simulink model "AerialManipulatorSystem"  (R2023b)
settings: Solver=FixedStepDiscrete  StartTime=0  StopTime=10  FixedStep=0.01  RelTol=1e-3
settings Model: Creator=Chen Fan  LastModifiedBy=Chen Fan
settings DataIOCC: ReturnWorkspaceOutputs=off

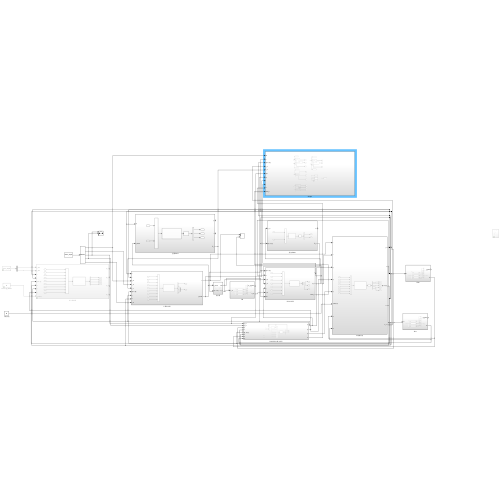
[thumbnail: Simulink's stored preview of the top-level diagram]
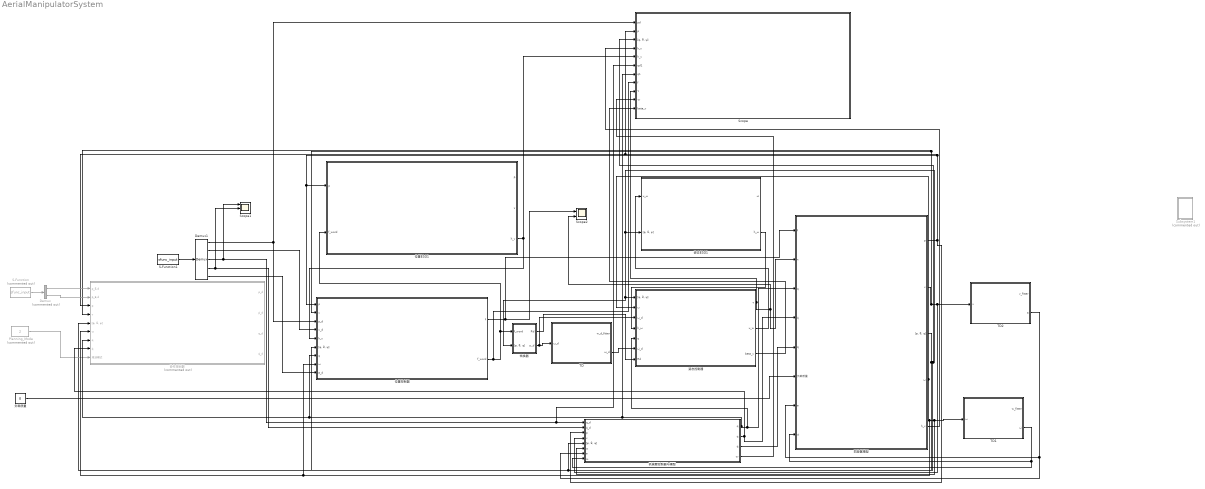
== system AerialManipulatorSystem ==
  Demux : Demux  Commented=on  Outputs=2
  Demux1 : Demux  Outputs=5
      settings: DisplayOption=none
  Planning_Mode : Constant  Commented=on  Value=2
  S-Function : S-Function  Commented=on  FunctionName=sfunc_input  SFunctionDeploymentMode=off  EnableBusSupport=off
  S-Function1 : S-Function  FunctionName=sfunc_input  SFunctionDeploymentMode=off  EnableBusSupport=off
  Scope : Subsystem
  Scope1 : Scope  NumInputPorts=3
  Scope2 : Scope  NumInputPorts=2
  Subsystem1 : Subsystem  Commented=on
  TD : Subsystem
  TD1 : Subsystem
  TD2 : Subsystem
  位置ESO1 : Subsystem
  位置控制器 : Subsystem
  协作规划器 : Subsystem  Commented=on
  四旋翼模型 : Subsystem
  姿态ESO1 : Subsystem
  姿态控制器 : Subsystem
  机械臂控制器与模型 : Subsystem
  负载质量 : Constant  Value=0
  转换器 : Subsystem
  wires:
  姿态控制器/1(τ) -> 四旋翼模型/2(τ), Scope2/2, Scope/9(τ)
  位置控制器/1(f) -> Scope2/1, 四旋翼模型/1(f)
  四旋翼模型/3("[φ, θ, ψ]") -> 位置控制器/6("[φ, θ, ψ]"), 机械臂控制器与模型/5("[φ, θ, ψ]"), 姿态ESO1/2("[φ, θ, ψ]"), 转换器/2("[φ, θ, ψ]"), 姿态控制器/1("[φ, θ, ψ]"), Scope/3("[φ, θ, ψ]"), 协作规划器/5("[φ, θ, ψ]")
  负载质量/1 -> 四旋翼模型/6(负载质量)
  四旋翼模型/1(p) -> 机械臂控制器与模型/3(p), 位置ESO1/1(p), 位置控制器/1(p), 协作规划器/3(p), Scope/2(p)
  Planning_Mode/1 -> 协作规划器/9(规划模式)
  机械臂控制器与模型/1(q) -> 姿态控制器/5(q), 四旋翼模型/3(q), Scope/7(q1), 位置控制器/7(q), 协作规划器/7(q)
  机械臂控制器与模型/2(q̇) -> 四旋翼模型/4(q̇), 协作规划器/8(q̇)
  机械臂控制器与模型/3(q̈) -> 四旋翼模型/5(q̈)
  四旋翼模型/4(ω) -> 协作规划器/6(ω), 位置控制器/8(ω), TD1/1(ω), 机械臂控制器与模型/6(ω), 姿态控制器/2(ω)
  四旋翼模型/2(v) -> TD2/1(v), 机械臂控制器与模型/4(v), 协作规划器/4(v), 位置控制器/2(v)
  S-Function/1 -> Demux/1
  Demux/1 -> 协作规划器/1(p_E,d)
  Demux/2 -> 协作规划器/2(ṗ_E,d)
  位置ESO1/3(ĥ_v) -> Scope/5(ĥ_v), 位置控制器/5(ĥ_v)
  姿态ESO1/2(ĥ_ω) -> 姿态控制器/4(ĥ_ω)
  TD/2(ω̇_d) -> 姿态控制器/6(ω̇_d)
  S-Function1/1 -> Demux1/1
  Demux1/4 -> Scope1/2, 机械臂控制器与模型/2(q̇_d)
  Demux1/3 -> Scope1/1, Scope/6(qd1), 机械臂控制器与模型/1(q_d)
  Demux1/1 -> Scope/1(pd), 位置控制器/3(p_d)
  Demux1/2 -> 位置控制器/4(v_d)
  TD1/2(ω̇) -> 机械臂控制器与模型/8(ω.), 四旋翼模型/8(ω̇)
  TD2/2(a) -> 机械臂控制器与模型/7(a), 四旋翼模型/7(a)
  Demux1/5 -> 位置控制器/9(a_d)
  转换器/2(ω_d) -> 姿态控制器/3(ω_d), TD/1(ω_d)
  转换器/1(Rd) -> 姿态控制器/7(Rd)
  位置控制器/2(f_word) -> Scope/8(f), 位置ESO1/2(f_word), 转换器/1(f_word)
  四旋翼模型/5(h_v) -> Scope/4(h_v)
  姿态控制器/2(u_w) -> 姿态ESO1/1(u_ω)
  机械臂控制器与模型/4(τr) -> Scope/10(τr)
  姿态控制器/3(beta_v) -> Scope/11(beta_v)

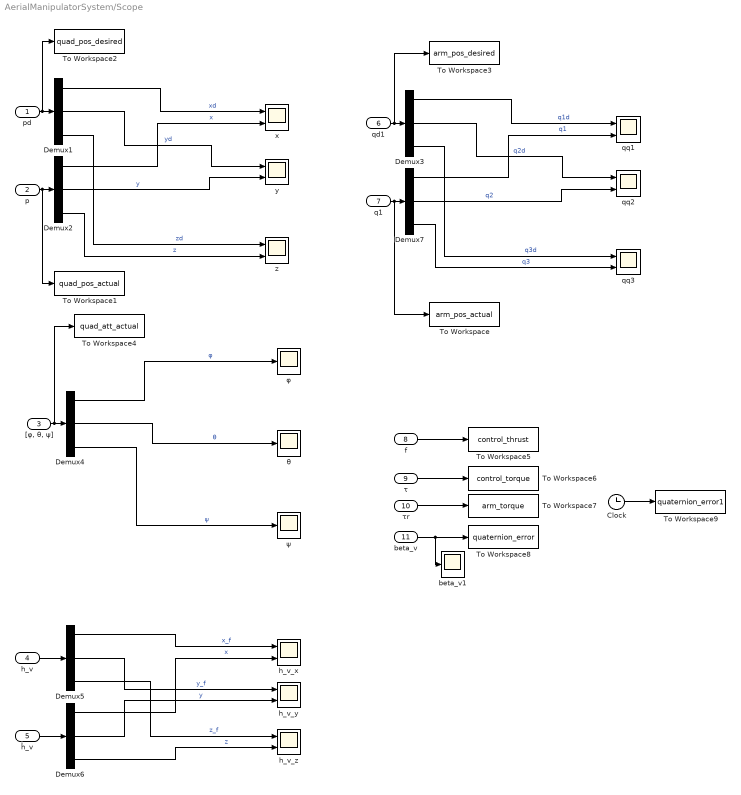
== system AerialManipulatorSystem/Scope ==
  pd : Inport
  p : Inport  Port=2
  "[φ, θ, ψ]" : Inport  Port=3
  h_v : Inport  Port=4
  ĥ_v : Inport  Port=5
  qd1 : Inport  Port=6
  q1 : Inport  Port=7
  f : Inport  Port=8
  τ : Inport  Port=9
  τr : Inport  Port=10
  beta_v : Inport  Port=11
  Clock : Clock
  Demux{1..7} (7 alike) : Demux  Outputs=3
  To Workspace : ToWorkspace  VariableName=arm_pos_actual  SaveFormat=Timeseries  SampleTime=-1
  To Workspace1 : ToWorkspace  VariableName=quad_pos_actual  SaveFormat=Timeseries  SampleTime=-1
  To Workspace2 : ToWorkspace  VariableName=quad_pos_desired  SaveFormat=Timeseries  SampleTime=-1
  To Workspace3 : ToWorkspace  VariableName=arm_pos_desired  SaveFormat=Timeseries  SampleTime=-1
  To Workspace4 : ToWorkspace  VariableName=quad_att_actual  SaveFormat=Timeseries  SampleTime=-1
  To Workspace5 : ToWorkspace  VariableName=control_thrust  SaveFormat=Timeseries  SampleTime=-1
  To Workspace6 : ToWorkspace  VariableName=control_torque  SaveFormat=Timeseries  SampleTime=-1
  To Workspace7 : ToWorkspace  VariableName=arm_torque  SaveFormat=Timeseries  SampleTime=-1
  To Workspace8 : ToWorkspace  VariableName=quaternion_error  SaveFormat=Timeseries  SampleTime=-1
  To Workspace9 : ToWorkspace  VariableName=quaternion_error1  SaveFormat=Timeseries  SampleTime=-1
  beta_v1 : Scope
  h_v_x : Scope  NumInputPorts=2
  h_v_y : Scope  NumInputPorts=2
  h_v_z : Scope  NumInputPorts=2
  qq1 : Scope  NumInputPorts=2
  qq2 : Scope  NumInputPorts=2
  qq3 : Scope  NumInputPorts=2
  x : Scope  NumInputPorts=2
  y : Scope  NumInputPorts=2
  z : Scope  NumInputPorts=2
  θ : Scope
  φ : Scope
  ψ : Scope
  wires:
  Demux2/3 -> z/2  "z"
  Demux4/3 -> ψ/1  "ψ"
  pd/1 -> To Workspace2/1, Demux1/1
  Demux1/1 -> x/1  "xd"
  p/1 -> To Workspace1/1, Demux2/1
  Demux2/2 -> y/2  "y"
  Demux2/1 -> x/2  "x"
  Demux1/2 -> y/1  "yd"
  Demux1/3 -> z/1  "zd"
  Demux4/2 -> θ/1  "θ"
  Demux4/1 -> φ/1  "φ"
  h_v/1 -> Demux5/1
  ĥ_v/1 -> Demux6/1
  Demux5/1 -> h_v_x/1  "x_f"
  Demux6/1 -> h_v_x/2  "x"
  Demux5/2 -> h_v_y/1  "y_f"
  Demux6/2 -> h_v_y/2  "y"
  Demux5/3 -> h_v_z/1  "z_f"
  Demux6/3 -> h_v_z/2  "z"
  Demux7/2 -> qq2/2  "q2"
  q1/1 -> To Workspace/1, Demux7/1
  Demux3/1 -> qq1/1  "q1d"
  qd1/1 -> To Workspace3/1, Demux3/1
  Demux3/2 -> qq2/1  "q2d"
  Demux7/3 -> qq3/2  "q3"
  Demux7/1 -> qq1/2  "q1"
  Demux3/3 -> qq3/1  "q3d"
  "[φ, θ, ψ]"/1 -> To Workspace4/1, Demux4/1
  f/1 -> To Workspace5/1
  τ/1 -> To Workspace6/1
  τr/1 -> To Workspace7/1
  beta_v/1 -> beta_v1/1, To Workspace8/1
  Clock/1 -> To Workspace9/1

== system AerialManipulatorSystem/Subsystem1 ==
  Arm_State_Delay : UnitDelay  Commented=on  InitialCondition=[0 0 0 0 0 0 0 0 0 0 0 0 0 0 0]  SampleTime=-1  HasFrameUpgradeWarning=on
  Attitude_Scope : Scope  Commented=on
  EndEffector_Data : ToWorkspace  Commented=on  VariableName=end_effector_data  SaveFormat=Timeseries  SampleTime=-1
  Position_Data : ToWorkspace  Commented=on  VariableName=position_data  SaveFormat=Timeseries  SampleTime=-1
  Position_Tracking_Scope : Scope  Commented=on  NumInputPorts=2
  Quad_State_Delay : UnitDelay  Commented=on  InitialCondition=[0 0 3 0 0 0 0 0 0 0 0 0]  SampleTime=-1  HasFrameUpgradeWarning=on
  Subsystem : Subsystem  Commented=on

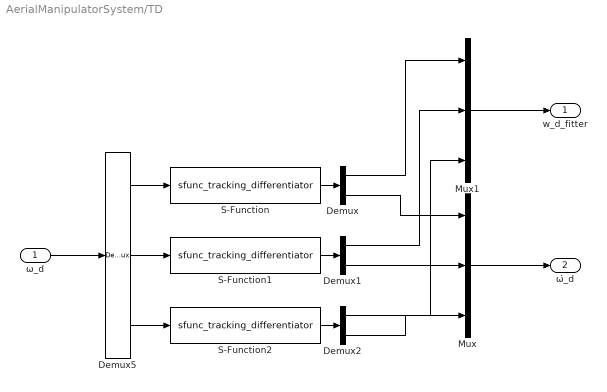
== system AerialManipulatorSystem/TD ==
  ω_d : Inport
  Demux : Demux  Outputs=2
  Demux1 : Demux  Outputs=2
  Demux2 : Demux  Outputs=2
  Demux5 : Demux  Outputs=3
  Mux : Mux  Inputs=3
  Mux1 : Mux  Inputs=3
  S-Function : S-Function  FunctionName=sfunc_tracking_differentiator  SFunctionDeploymentMode=off  EnableBusSupport=off
  S-Function1 : S-Function  FunctionName=sfunc_tracking_differentiator  SFunctionDeploymentMode=off  EnableBusSupport=off
  S-Function2 : S-Function  FunctionName=sfunc_tracking_differentiator  SFunctionDeploymentMode=off  EnableBusSupport=off
  w_d_fitter : Outport
  ω̇_d : Outport  Port=2
  wires:
  Demux5/2 -> S-Function1/1
  Demux5/1 -> S-Function/1
  ω_d/1 -> Demux5/1
  S-Function/1 -> Demux/1
  S-Function1/1 -> Demux1/1
  Demux/2 -> Mux/1
  Demux1/2 -> Mux/2
  Demux5/3 -> S-Function2/1
  S-Function2/1 -> Demux2/1
  Demux2/2 -> Mux/3
  Demux/1 -> Mux1/1
  Demux1/1 -> Mux1/2
  Demux2/1 -> Mux1/3
  Mux/1 -> ω̇_d/1
  Mux1/1 -> w_d_fitter/1

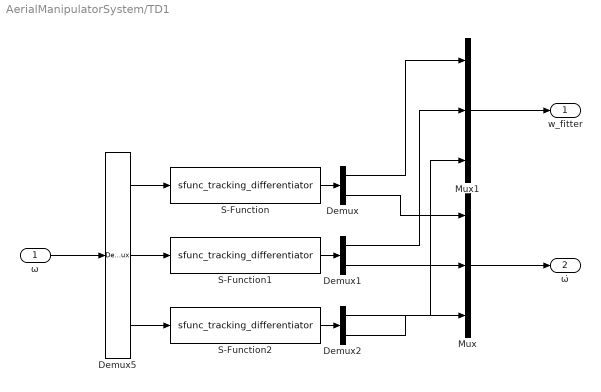
== system AerialManipulatorSystem/TD1 ==
  ω : Inport
  Demux : Demux  Outputs=2
  Demux1 : Demux  Outputs=2
  Demux2 : Demux  Outputs=2
  Demux5 : Demux  Outputs=3
  Mux : Mux  Inputs=3
  Mux1 : Mux  Inputs=3
  S-Function : S-Function  FunctionName=sfunc_tracking_differentiator  SFunctionDeploymentMode=off  EnableBusSupport=off
  S-Function1 : S-Function  FunctionName=sfunc_tracking_differentiator  SFunctionDeploymentMode=off  EnableBusSupport=off
  S-Function2 : S-Function  FunctionName=sfunc_tracking_differentiator  SFunctionDeploymentMode=off  EnableBusSupport=off
  w_fitter : Outport
  ω̇ : Outport  Port=2
  wires:
  Demux5/2 -> S-Function1/1
  Demux5/1 -> S-Function/1
  ω/1 -> Demux5/1
  S-Function/1 -> Demux/1
  S-Function1/1 -> Demux1/1
  Demux/2 -> Mux/1
  Demux1/2 -> Mux/2
  Demux5/3 -> S-Function2/1
  S-Function2/1 -> Demux2/1
  Demux2/2 -> Mux/3
  Demux/1 -> Mux1/1
  Demux1/1 -> Mux1/2
  Demux2/1 -> Mux1/3
  Mux/1 -> ω̇/1
  Mux1/1 -> w_fitter/1

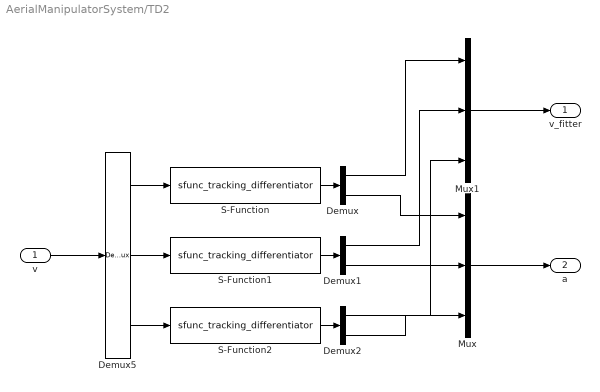
== system AerialManipulatorSystem/TD2 ==
  v : Inport
  Demux : Demux  Outputs=2
  Demux1 : Demux  Outputs=2
  Demux2 : Demux  Outputs=2
  Demux5 : Demux  Outputs=3
  Mux : Mux  Inputs=3
  Mux1 : Mux  Inputs=3
  S-Function : S-Function  FunctionName=sfunc_tracking_differentiator  SFunctionDeploymentMode=off  EnableBusSupport=off
  S-Function1 : S-Function  FunctionName=sfunc_tracking_differentiator  SFunctionDeploymentMode=off  EnableBusSupport=off
  S-Function2 : S-Function  FunctionName=sfunc_tracking_differentiator  SFunctionDeploymentMode=off  EnableBusSupport=off
  v_fitter : Outport
  a : Outport  Port=2
  wires:
  Demux5/2 -> S-Function1/1
  Demux5/1 -> S-Function/1
  v/1 -> Demux5/1
  S-Function/1 -> Demux/1
  S-Function1/1 -> Demux1/1
  Demux/2 -> Mux/1
  Demux1/2 -> Mux/2
  Demux5/3 -> S-Function2/1
  S-Function2/1 -> Demux2/1
  Demux2/2 -> Mux/3
  Demux/1 -> Mux1/1
  Demux1/1 -> Mux1/2
  Demux2/1 -> Mux1/3
  Mux/1 -> a/1
  Mux1/1 -> v_fitter/1

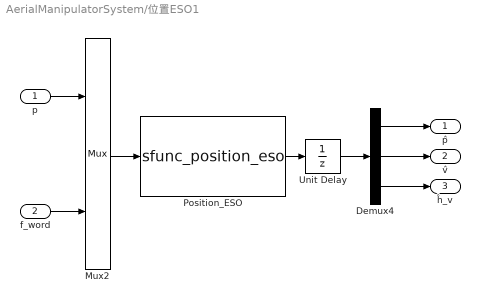
== system AerialManipulatorSystem/位置ESO1 ==
  p : Inport
  f_word : Inport  Port=2
  Demux4 : Demux  Outputs=3
  Mux2 : Mux  Inputs=2
  Position_ESO : S-Function  FunctionName=sfunc_position_eso  SFunctionDeploymentMode=off  EnableBusSupport=off
  Unit Delay : UnitDelay  SampleTime=-1  HasFrameUpgradeWarning=on
  p̂ : Outport
  v̂ : Outport  Port=2
  ĥ_v : Outport  Port=3
  wires:
  p/1 -> Mux2/1
  Position_ESO/1 -> Unit Delay/1
  Demux4/2 -> v̂/1
  Mux2/1 -> Position_ESO/1
  Demux4/3 -> ĥ_v/1
  Demux4/1 -> p̂/1
  f_word/1 -> Mux2/2
  Unit Delay/1 -> Demux4/1

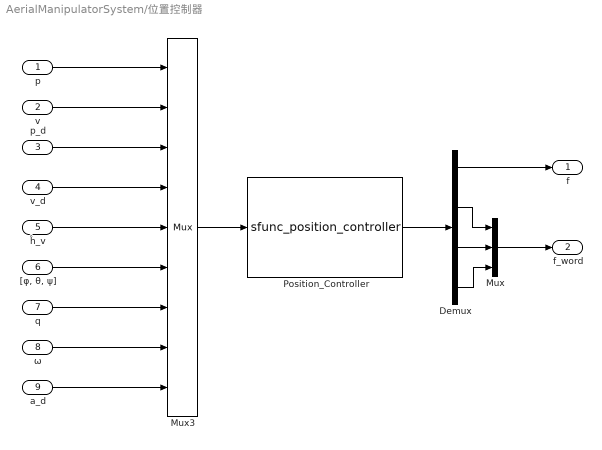
== system AerialManipulatorSystem/位置控制器 ==
  p : Inport
  v : Inport  Port=2
  p_d : Inport  Port=3
  v_d : Inport  Port=4
  ĥ_v : Inport  Port=5
  "[φ, θ, ψ]" : Inport  Port=6
  q : Inport  Port=7
  ω : Inport  Port=8
  a_d : Inport  Port=9
  Demux : Demux
  Mux : Mux  Inputs=3
  Mux3 : Mux  Inputs=9
  Position_Controller : S-Function  FunctionName=sfunc_position_controller  SFunctionDeploymentMode=off  EnableBusSupport=off
  f : Outport
  f_word : Outport  Port=2
  wires:
  Mux3/1 -> Position_Controller/1
  p/1 -> Mux3/1
  Position_Controller/1 -> Demux/1
  v_d/1 -> Mux3/4
  ĥ_v/1 -> Mux3/5
  v/1 -> Mux3/2
  p_d/1 -> Mux3/3
  "[φ, θ, ψ]"/1 -> Mux3/6
  q/1 -> Mux3/7
  Demux/1 -> f/1
  Demux/2 -> Mux/1
  Demux/3 -> Mux/2
  Demux/4 -> Mux/3
  Mux/1 -> f_word/1
  ω/1 -> Mux3/8
  a_d/1 -> Mux3/9

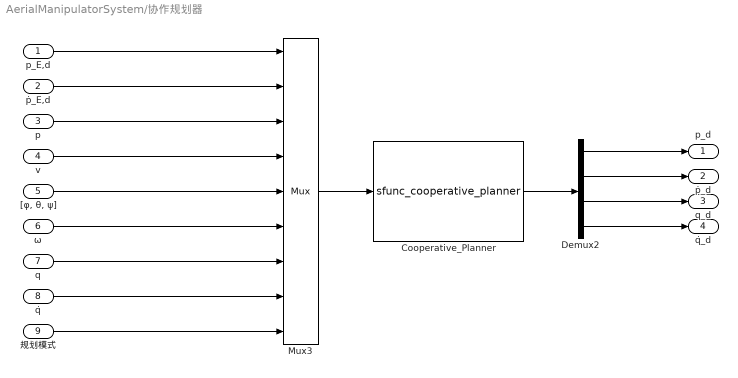
== system AerialManipulatorSystem/协作规划器 ==
  p_E,d : Inport
  ṗ_E,d : Inport  Port=2
  p : Inport  Port=3
  v : Inport  Port=4
  "[φ, θ, ψ]" : Inport  Port=5
  ω : Inport  Port=6
  q : Inport  Port=7
  q̇ : Inport  Port=8
  规划模式 : Inport  Port=9
  Cooperative_Planner : S-Function  FunctionName=sfunc_cooperative_planner  SFunctionDeploymentMode=off  EnableBusSupport=off
  Demux2 : Demux
  Mux3 : Mux  Inputs=9
  p_d : Outport
  ṗ_d : Outport  Port=2
  q_d : Outport  Port=3
  q̇_d : Outport  Port=4
  wires:
  ω/1 -> Mux3/6
  Demux2/3 -> q_d/1
  Cooperative_Planner/1 -> Demux2/1
  Demux2/4 -> q̇_d/1
  "[φ, θ, ψ]"/1 -> Mux3/5
  Mux3/1 -> Cooperative_Planner/1
  v/1 -> Mux3/4
  q/1 -> Mux3/7
  q̇/1 -> Mux3/8
  p/1 -> Mux3/3
  ṗ_E,d/1 -> Mux3/2
  规划模式/1 -> Mux3/9
  p_E,d/1 -> Mux3/1
  Demux2/1 -> p_d/1
  Demux2/2 -> ṗ_d/1

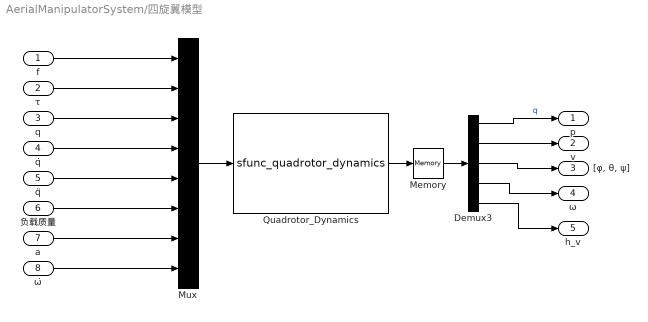
== system AerialManipulatorSystem/四旋翼模型 ==
  f : Inport
  τ : Inport  Port=2
  q : Inport  Port=3
  q̇ : Inport  Port=4
  q̈ : Inport  Port=5
  负载质量 : Inport  Port=6
  a : Inport  Port=7
  ω̇ : Inport  Port=8
  Demux3 : Demux  Outputs=5
  Memory : Memory  InitialCondition=[0 0 5 0 0 0 0 0 0 0 0 0 0 0 0]  InheritSampleTime=on
  Mux : Mux  Inputs=8
  Quadrotor_Dynamics : S-Function  FunctionName=sfunc_quadrotor_dynamics  SFunctionDeploymentMode=off  EnableBusSupport=off
  p : Outport
  v : Outport  Port=2
  "[φ, θ, ψ]" : Outport  Port=3
  ω : Outport  Port=4
  h_v : Outport  Port=5
  wires:
  负载质量/1 -> Mux/6
  Mux/1 -> Quadrotor_Dynamics/1
  q/1 -> Mux/3
  q̈/1 -> Mux/5
  Demux3/1 -> p/1  "q"
  Demux3/3 -> "[φ, θ, ψ]"/1
  q̇/1 -> Mux/4
  Demux3/2 -> v/1
  Demux3/4 -> ω/1
  τ/1 -> Mux/2
  f/1 -> Mux/1
  Quadrotor_Dynamics/1 -> Memory/1
  Memory/1 -> Demux3/1
  a/1 -> Mux/7
  ω̇/1 -> Mux/8
  Demux3/5 -> h_v/1

== system AerialManipulatorSystem/姿态ESO1 ==
  u_ω : Inport
  "[φ, θ, ψ]" : Inport  Port=2
  Attitude_ESO : S-Function  FunctionName=sfunc_attitude_eso  SFunctionDeploymentMode=off  EnableBusSupport=off
  Demux4 : Demux  Outputs=2
  Mux3 : Mux  Inputs=2
  Unit Delay1 : UnitDelay  SampleTime=-1  HasFrameUpgradeWarning=on
  "ω̂ " : Outport
  ĥ_ω : Outport  Port=2
  wires:
  Attitude_ESO/1 -> Unit Delay1/1
  Demux4/2 -> ĥ_ω/1  "q̇"
  Mux3/1 -> Attitude_ESO/1
  Demux4/1 -> "ω̂ "/1  "q"
  Unit Delay1/1 -> Demux4/1
  u_ω/1 -> Mux3/1
  "[φ, θ, ψ]"/1 -> Mux3/2

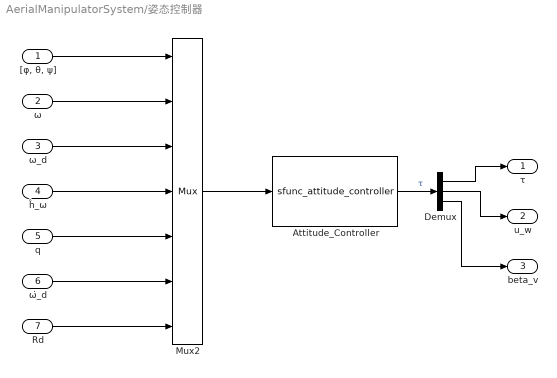
== system AerialManipulatorSystem/姿态控制器 ==
  "[φ, θ, ψ]" : Inport
  ω : Inport  Port=2
  ω_d : Inport  Port=3
  ĥ_ω : Inport  Port=4
  q : Inport  Port=5
  ω̇_d : Inport  Port=6
  Rd : Inport  Port=7
  Attitude_Controller : S-Function  FunctionName=sfunc_attitude_controller  SFunctionDeploymentMode=off  EnableBusSupport=off
  Demux : Demux  Outputs=3
  Mux2 : Mux  Inputs=7
  τ : Outport
  u_w : Outport  Port=2
  beta_v : Outport  Port=3
  wires:
  "[φ, θ, ψ]"/1 -> Mux2/1
  ω/1 -> Mux2/2
  Mux2/1 -> Attitude_Controller/1
  Rd/1 -> Mux2/7
  ω̇_d/1 -> Mux2/6
  q/1 -> Mux2/5
  ĥ_ω/1 -> Mux2/4
  ω_d/1 -> Mux2/3
  Attitude_Controller/1 -> Demux/1  "τ"
  Demux/1 -> τ/1
  Demux/2 -> u_w/1
  Demux/3 -> beta_v/1

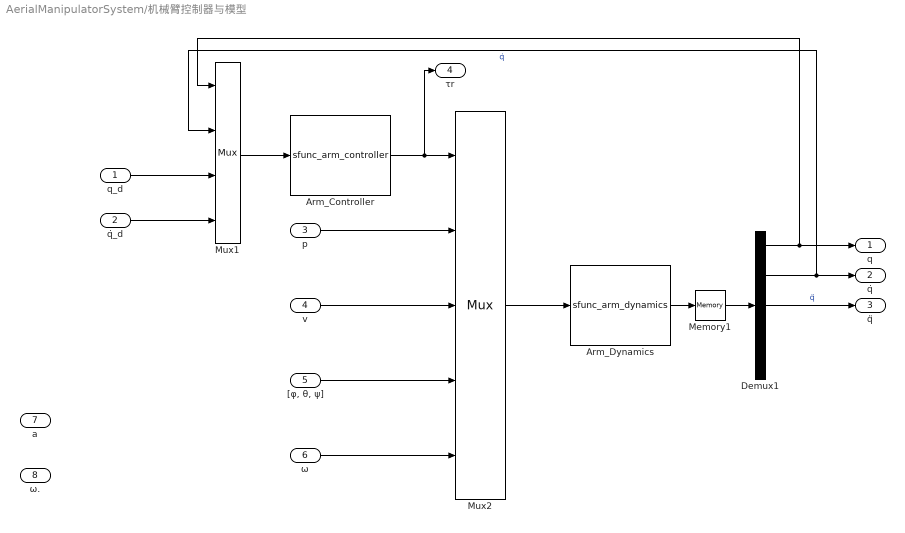
== system AerialManipulatorSystem/机械臂控制器与模型 ==
  q_d : Inport
  q̇_d : Inport  Port=2
  p : Inport  Port=3
  v : Inport  Port=4
  "[φ, θ, ψ]" : Inport  Port=5
  ω : Inport  Port=6
  a : Inport  Port=7
  ω. : Inport  Port=8
  Arm_Controller : S-Function  FunctionName=sfunc_arm_controller  SFunctionDeploymentMode=off  EnableBusSupport=off
  Arm_Dynamics : S-Function  FunctionName=sfunc_arm_dynamics  SFunctionDeploymentMode=off  EnableBusSupport=off
  Demux1 : Demux  Outputs=5
  Memory1 : Memory  InheritSampleTime=on
  Mux1 : Mux
  Mux2 : Mux  Inputs=5
  q : Outport
  q̇ : Outport  Port=2
  q̈ : Outport  Port=3
  τr : Outport  Port=4
  wires:
  Demux1/3 -> q̈/1  "q̈"
  Demux1/2 -> Mux1/2, q̇/1  "q̇"
  Arm_Dynamics/1 -> Memory1/1
  Demux1/1 -> Mux1/1, q/1
  Mux1/1 -> Arm_Controller/1
  q_d/1 -> Mux1/3
  q̇_d/1 -> Mux1/4
  Arm_Controller/1 -> τr/1, Mux2/1
  Mux2/1 -> Arm_Dynamics/1
  p/1 -> Mux2/2
  v/1 -> Mux2/3
  "[φ, θ, ψ]"/1 -> Mux2/4
  ω/1 -> Mux2/5
  Memory1/1 -> Demux1/1

== system AerialManipulatorSystem/转换器 ==
  f_word : Inport
  "[φ, θ, ψ]" : Inport  Port=2
  Demux2 : Demux
  Mux : Mux  Inputs=2
  Mux1 : Mux  Inputs=3
  S-Function2 : S-Function  FunctionName=sfunc_Tranformation  SFunctionDeploymentMode=off  EnableBusSupport=off
  Rd : Outport
  ω_d : Outport  Port=2
  wires:
  S-Function2/1 -> Demux2/1
  Mux/1 -> S-Function2/1
  f_word/1 -> Mux/1
  "[φ, θ, ψ]"/1 -> Mux/2
  Demux2/4 -> ω_d/1
  Demux2/1 -> Mux1/1
  Demux2/2 -> Mux1/2
  Demux2/3 -> Mux1/3
  Mux1/1 -> Rd/1

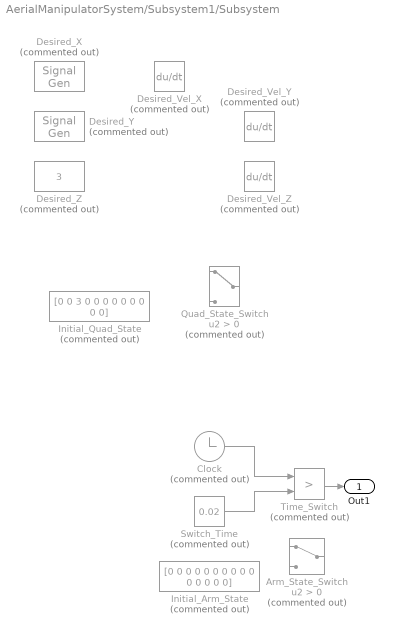
== system AerialManipulatorSystem/Subsystem1/Subsystem ==
  Arm_State_Switch : Switch  Commented=on  Criteria=u2 > Threshold  SaturateOnIntegerOverflow=off  InputSameDT=off
  Clock : Clock  Commented=on
  Desired_Vel_X : Derivative  Commented=on
  Desired_Vel_Y : Derivative  Commented=on
  Desired_Vel_Z : Derivative  Commented=on
  Desired_X : SignalGenerator  Commented=on  Amplitude=1.5  Frequency=0.1  Units=rad/sec
  Desired_Y : SignalGenerator  Commented=on  Amplitude=1.5  Frequency=0.1  Units=rad/sec
  Desired_Z : Constant  Commented=on  Value=3
  Initial_Arm_State : Constant  Commented=on  Value=[0 0 0 0 0 0 0 0 0 0 0 0 0 0 0]
  Initial_Quad_State : Constant  Commented=on  Value=[0 0 3 0 0 0 0 0 0 0 0 0]
  Quad_State_Switch : Switch  Commented=on  Criteria=u2 > Threshold  SaturateOnIntegerOverflow=off  InputSameDT=off
  Switch_Time : Constant  Commented=on  Value=0.02
  Time_Switch : RelationalOperator  Commented=on  Operator=>  OutDataTypeStr=boolean  RndMeth=Simplest  InputSameDT=off
  Out1 : Outport
  wires:
  Time_Switch/1 -> Out1/1
  Clock/1 -> Time_Switch/1
  Switch_Time/1 -> Time_Switch/2
